simulink model "week1_8"  (R2020b)
settings: Solver=VariableStepAuto  StartTime=0.0  StopTime=inf  RelTol=1e-3
settings Model: Creator=HP  LastModifiedBy=HP

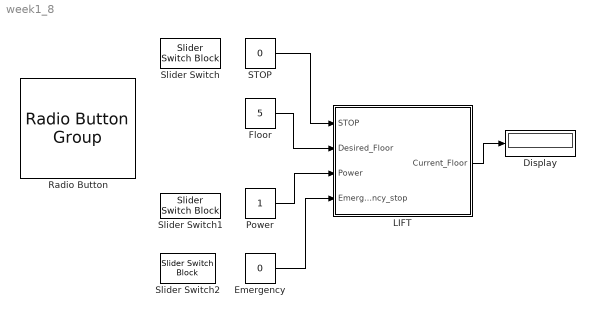
== system week1_8 ==
  Display : Display
  Emergency : Constant  Value=0
  Floor : Constant  Value=5
  "LIFT " : Stateflow chart  TreatAsAtomicUnit=on
  Power : Constant
  Radio Button : RadioButtonGroup  LabelPosition=Bottom  SelectedLabel=Fifth Floor  ButtonGroupName=Group
      settings: Values={{'First  Floor', 'Second Floor', 'Third Floor', 'Fourth Floor', 'Fifth Floor'}, [1 2 3 4 5]}
  STOP : Constant  Value=0
  Slider Switch : SliderSwitchBlock
      settings: Values={{'Off', 'On'}, [0 1]}
  Slider Switch1 : SliderSwitchBlock
      settings: Values={{'Off', 'On'}, [0 1]}
  Slider Switch2 : SliderSwitchBlock
      settings: Values={{'Off', 'On'}, [0 1]}
  wires:
  STOP/1 -> "LIFT "/1(STOP)
  "LIFT "/1(Current_Floor) -> Display/1
  Floor/1 -> "LIFT "/2(Desired_Floor)
  Power/1 -> "LIFT "/3(Power)
  Emergency/1 -> "LIFT "/4(Emergency_stop)

== stateflow chart week1_8/LIFT  ==
  state Lift [parallel]
    settings: executionOrder=1
    (history)
    state Power
    state NORMAL
      state Loop1 [parallel]
        settings: executionOrder=1
        (history)
        state Emer
          en:
        state Loop2
          state Fan_Light [parallel]
            settings: executionOrder=2
            (history)
            state Fan_Light_Off
            state Fan_Light_On
            (default) -> Fan_Light_Off
            Fan_Light_Off -> Fan_Light_On : On{disp 'Fan and Light are On'}
            Fan_Light_On -> Fan_Light_Off : Off{disp 'Fan and Light are OFF'}
          state Working [parallel]
            en:
            disp 'LIFT RUNNING';
            settings: executionOrder=1
            (history)
            state Off
              en:
              disp 'LIFT STOPPED';
            state On
              en:
              (history)
              state First
                entry:
                i=1;
                Current_Floor=1;
                disp '1 Floor';
              state Second
                en:
                i=2;
                Current_Floor=2;
                disp '2 Floor';
              state Third
                en:
                i=3;
                Current_Floor=3;
                disp '3 Floor';
              state Fifth
                en:
                i=5;
                Current_Floor=5;
                disp '5 Floor';
              state Fourth
                en:
                i=4;
                Current_Floor=4;
                disp '4 Floor';
              (default) -> First
              Second -> Third [order 2] : [i<Desired_Floor]
              Third -> Fourth [order 1] : [i<Desired_Floor]
              Fourth -> Fifth [order 1] : [i<Desired_Floor]
              First -> Second : [i<Desired_Floor]
              Fifth -> Fourth : [i>Desired_Floor]
              Fourth -> Third [order 2] : [i>Desired_Floor]
              Second -> First [order 1] : [i>Desired_Floor]
              Third -> Second [order 2] : [i>Desired_Floor]
            (default) -> Off
            Off -> On : [STOP==0]{send(On,Fan_Light)}
            On -> Off : [STOP==1]{send(Off,Fan_Light)}
        (default) -> Emer
        Emer -> Loop2 : [Emergency_stop==0]{send(No_emg,Emergency)}
        Loop2 -> Emer : [Emergency_stop==1]{send(Emg,Emergency)}
      state Emergency [parallel]
        settings: executionOrder=2
        (history)
        state Emg_off
          en:
        state Emg_On
          en:
          disp 'EMERGENCY STOP AND ALARM ARE ON';
        (default) -> Emg_off
        Emg_off -> Emg_On : Emg
        Emg_On -> Emg_off : No_emg{disp 'EMERGENCY STOP AND ALARM ARE OFF'}
    (default) -> Power
    Power -> NORMAL : [Power==1]{disp 'Power On'}
    NORMAL -> Power : [Power==0]{disp 'Power Off'}
  data: i local; STOP input; Current_Floor output; Desired_Floor input; Power input; Emergency_stop input
  events: Emg local FUNCTION_CALL_EVENT; No_emg local FUNCTION_CALL_EVENT; Off local FUNCTION_CALL_EVENT; On local FUNCTION_CALL_EVENT
